simulink model "AAI"  (R2023a)
settings: Solver=FixedStepAuto  StartTime=0.0  StopTime=10.0  FixedStep=1e-3  RelTol=1e-3  EnableMultiTasking=on
settings Model: ExtModeTrigDuration=5  Creator=tstic  LastModifiedBy=nehac
settings OptimizationCC: EnhancedBackFolding=on  PassReuseOutputArgsAs=Individual arguments  ZeroExternalMemoryAtStartup=off  ZeroInternalMemoryAtStartup=off  MaxStackSize=64  OptimizeBlockOrder=speed  DifferentSizesBufferReuse=on  OptimizationCustomize=off  EfficientTunableParamExpr=on
settings DebuggingCC: ParameterTunabilityLossMsg=error
settings HardwareCC: ProdBitPerPointer=32  ProdBitPerSizeT=32  ProdBitPerPtrDiffT=32  ProdLargestAtomicInteger=Long  ProdLargestAtomicFloat=Double  ProdWordSize=32  ProdHWDeviceType=ARM Compatible->ARM Cortex
settings SFSimCC: MATLABDynamicMemAlloc=off
settings RTWCC: Description=Embedded Coder  SystemTargetFile=ert.tlc  HardwareBoard=NXP FRDM-K64F  TLCOptions="-aInlineSetEventsForThisBaseRateFcn=TLC_FALSE -aSuppressMultiTaskScheduler=TLC_FALSE  -aRateBasedStepFcn=0"  TemplateMakefile=ert_default_tmf  Toolchain=GNU Tools for ARM Embedded Processors
settings CodeAppCC: ForceParamTrailComments=on  IgnoreCustomStorageClasses=off  OperatorAnnotations=on  SimulinkDataObjDesc=on  SFDataObjDesc=on  InsertBlockDesc=on
settings ERTTargetCC: ExtModeTransport=4  ExtModeMexFile=sendToCommService

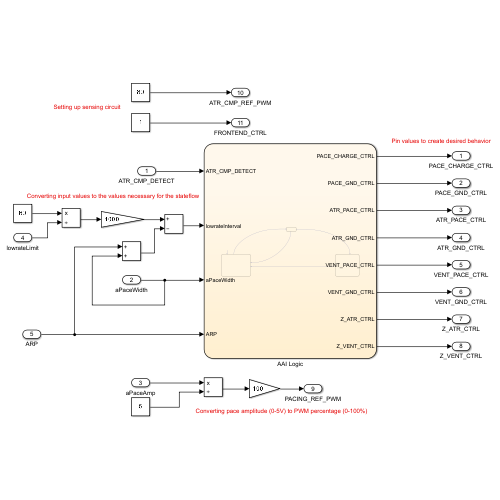
[thumbnail: Simulink's stored preview of the top-level diagram]
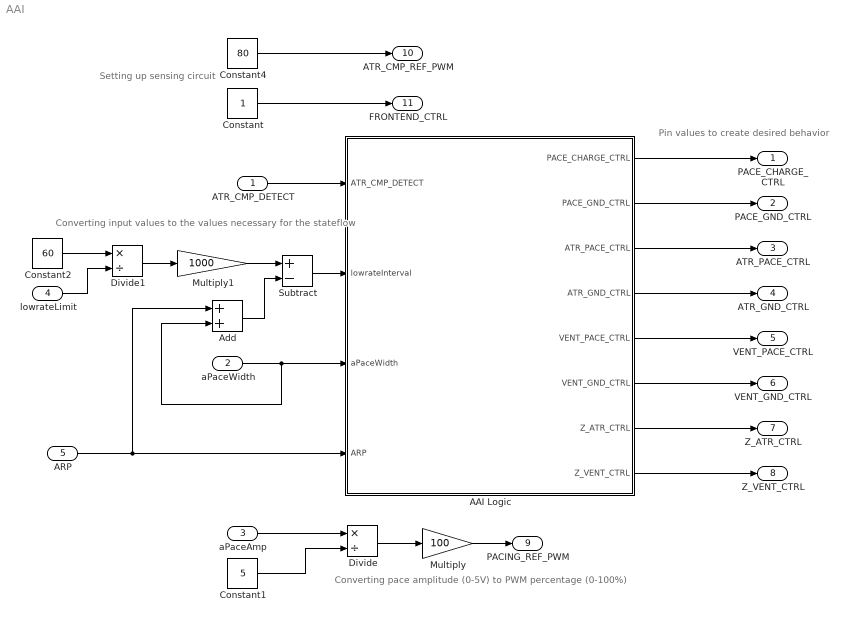
== system AAI ==
  note: Converting input values to the values necessary for the stateflow
  note: Converting pace amplitude (0-5V) to PWM percentage (0-100%)
  note: Pin values to create desired behavior
  note: Setting up sensing circuit
  ATR_CMP_DETECT : Inport  OutDataTypeStr=boolean
  aPaceWidth : Inport  Port=2
  aPaceAmp : Inport  Port=3
  lowrateLimit : Inport  Port=4
  ARP : Inport  Port=5
  AAI Logic : Stateflow chart  TreatAsAtomicUnit=on
  Add : Sum
  Constant : Constant
  Constant1 : Constant  Value=5
  Constant2 : Constant  Value=60
  Constant4 : Constant  Value=80
  Divide : Product  Inputs=*/
  Divide1 : Product  Inputs=*/
  Multiply : Gain  Gain=100
  Multiply1 : Gain  Gain=1000
  Subtract : Sum  Inputs=+-
  PACE_CHARGE_CTRL : Outport
  PACE_GND_CTRL : Outport  Port=2
  ATR_PACE_CTRL : Outport  Port=3
  ATR_GND_CTRL : Outport  Port=4
  VENT_PACE_CTRL : Outport  Port=5
  VENT_GND_CTRL : Outport  Port=6
  Z_ATR_CTRL : Outport  Port=7
  Z_VENT_CTRL : Outport  Port=8
  PACING_REF_PWM : Outport  Port=9
  ATR_CMP_REF_PWM : Outport  Port=10
  FRONTEND_CTRL : Outport  Port=11
  wires:
  Constant4/1 -> ATR_CMP_REF_PWM/1
  Constant1/1 -> Divide/2
  aPaceAmp/1 -> Divide/1
  Constant/1 -> FRONTEND_CTRL/1
  ATR_CMP_DETECT/1 -> AAI Logic/1(ATR_CMP_DETECT)
  ARP/1 -> Add/1, AAI Logic/4(ARP)
  aPaceWidth/1 -> AAI Logic/3(aPaceWidth), Add/2
  AAI Logic/1(PACE_CHARGE_CTRL) -> PACE_CHARGE_CTRL/1
  AAI Logic/2(PACE_GND_CTRL) -> PACE_GND_CTRL/1
  AAI Logic/3(ATR_PACE_CTRL) -> ATR_PACE_CTRL/1
  AAI Logic/4(ATR_GND_CTRL) -> ATR_GND_CTRL/1
  AAI Logic/5(VENT_PACE_CTRL) -> VENT_PACE_CTRL/1
  AAI Logic/6(VENT_GND_CTRL) -> VENT_GND_CTRL/1
  AAI Logic/7(Z_ATR_CTRL) -> Z_ATR_CTRL/1
  AAI Logic/8(Z_VENT_CTRL) -> Z_VENT_CTRL/1
  Divide/1 -> Multiply/1
  Multiply/1 -> PACING_REF_PWM/1
  Divide1/1 -> Multiply1/1
  Multiply1/1 -> Subtract/1
  Add/1 -> Subtract/2
  Subtract/1 -> AAI Logic/2(lowrateInterval)
  lowrateLimit/1 -> Divide1/2
  Constant2/1 -> Divide1/1

== stateflow chart AAI/AAI Logic ==
  note: After the ARP has passed, stay in this state until an atrial event is sensed or the low rate interval has passed
  state Sensing
  state Charging
    entry:
    PACE_GND_CTRL = 1;
    ATR_PACE_CTRL = 0;
    Z_ATR_CTRL = 0;
    Z_VENT_CTRL = 0;
    VENT_PACE_CTRL = 0;
    VENT_GND_CTRL = 0;
    ATR_GND_CTRL = 1;
    during:
    PACE_CHARGE_CTRL = 1;
  state Pacing
    entry:
    PACE_CHARGE_CTRL = 0;
    PACE_GND_CTRL = 1;
    VENT_PACE_CTRL = 0;
    VENT_GND_CTRL = 0;
    Z_VENT_CTRL = 0;
    Z_ATR_CTRL = 0;
    ATR_GND_CTRL = 0;
    ATR_PACE_CTRL = 1;
  note: Pin configuration for charging C22 and discharging C21
  note: Pin configuration for discharging C21 into the heart
  Charging -> Sensing : [after(ARP,msec)]
  Sensing -> Pacing [order 1] : [after(lowrateInterval,msec)]
  Sensing -> Charging [order 2] : [ATR_CMP_DETECT]
  (default) -> Charging
  Pacing -> Charging : [after(aPaceWidth,msec)]
  data: ATR_CMP_DETECT input; PACE_CHARGE_CTRL output; PACE_GND_CTRL output; ATR_PACE_CTRL output; ATR_GND_CTRL output; VENT_PACE_CTRL output; VENT_GND_CTRL output; Z_ATR_CTRL output; Z_VENT_CTRL output; lowrateInterval input; aPaceWidth input; ARP input; noPulseIn local [0..] =0
